simulink model "SeparacionJoystick"  (R2020b)
settings: Solver=VariableStepAuto  StartTime=0.0  StopTime=10  RelTol=1e-3
libraries: vrlib x1
settings Model: Creator=Jesus  LastModifiedBy=Jesus

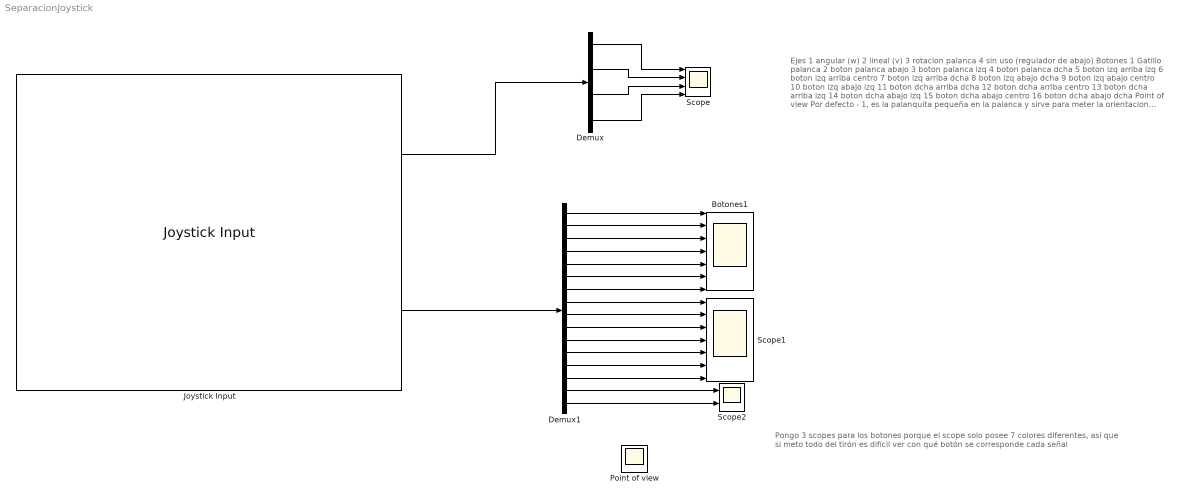
== system SeparacionJoystick ==
  note: Pongo 3 scopes para los botones porque el scope solo posee 7 colores diferentes,
      | así que si meto todo del tirón es difícil ver con qué botón se corresponde cada señal
  note: Ejes
      | 1 angular (w)
      | 2 lineal (v)
      | 3 rotacion palanca
      | 4 sin uso (regulador de abajo)
      |
      | Botones
      | 1 Gatillo palanca
      | 2 boton palanca abajo
      | 3 boton palanca izq
      | 4 boton palanca dcha
      | 5 boton izq arriba izq
      | 6 boton izq arriba centro
      | 7 boton izq arriba dcha
      | 8 boton izq abajo dcha
      | 9 boton izq abajo centro
      | 10 boton izq abajo izq
      | 11 boton dcha arriba dcha
      | 12 boton dcha arriba centro
      | 13 boton dcha arriba izq
      | 14 boton dcha abajo izq
      | 15 boton dcha abajo centro
      | 16 boton dcha abajo dcha
      |
      | Point of view
      | Por defecto - 1, es la palanquita pequeña en la palanca y sirve para meter la orientacion que queramos (entre 0 y 360)
  Botones1 : Scope  NumInputPorts=7
  Demux : Demux
  Demux1 : Demux  Outputs=16
  Joystick Input : vrlib/Joystick Input  joyid=1  adjustports=on  forcefeed=off
  Point of view : Scope
  Scope : Scope  NumInputPorts=4
  Scope1 : Scope  NumInputPorts=7
  Scope2 : Scope  NumInputPorts=2
  wires:
  Joystick Input/1 -> Demux/1
  Demux/1 -> Scope/1
  Demux/2 -> Scope/2
  Demux/3 -> Scope/3
  Demux/4 -> Scope/4
  ? -> Point of view/1
  Joystick Input/2 -> Demux1/1
  Demux1/1 -> Botones1/1
  Demux1/2 -> Botones1/2
  Demux1/3 -> Botones1/3
  Demux1/4 -> Botones1/4
  Demux1/5 -> Botones1/5
  Demux1/6 -> Botones1/6
  Demux1/7 -> Botones1/7
  Demux1/8 -> Scope1/1
  Demux1/9 -> Scope1/2
  Demux1/10 -> Scope1/3
  Demux1/11 -> Scope1/4
  Demux1/12 -> Scope1/5
  Demux1/13 -> Scope1/6
  Demux1/14 -> Scope1/7
  Demux1/16 -> Scope2/2
  Demux1/15 -> Scope2/1
